simulink model "intelligent_vehicle_example2"  (R2017a)
settings: Solver=VariableStepAuto  StartTime=0.0  StopTime=10.0  RelTol=1e-3
undefined symbols (not defined in the file or in its folder): b1, b2, K1, K2, M1, M2
settings Model: Creator=edward  LastModifiedBy=edward

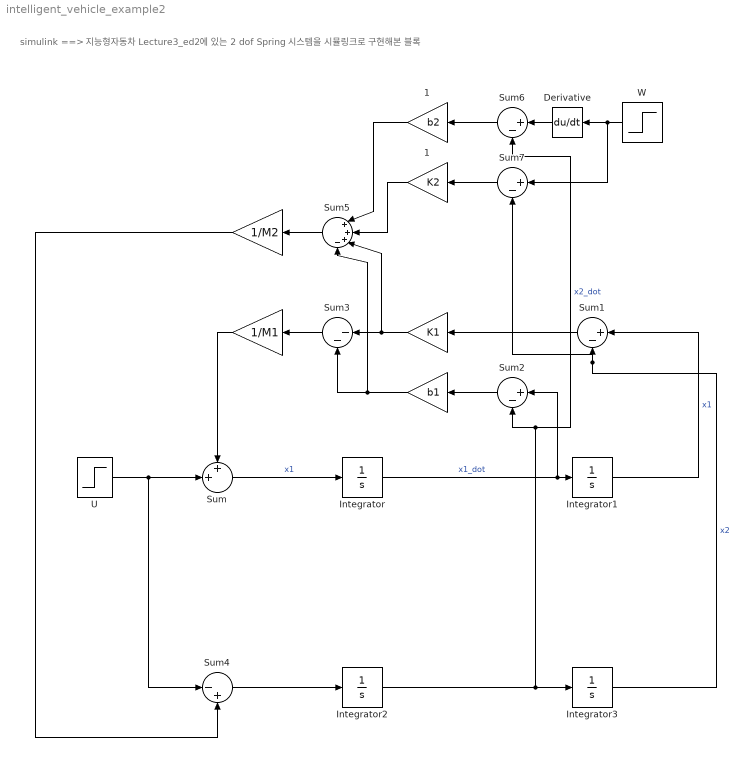
== system intelligent_vehicle_example2 ==
  note: simulink ==> 지능형자동차 Lecture3_ed2에 있는 2 dof Spring 시스템을 시뮬링크로 구현해본 블록
  " " : Gain  Gain=1/M2
  "  " : Gain  Gain=1/M1
  "   " : Gain  Gain=K1
  "    " : Gain  Gain=b1
  "    1" : Gain  Gain=b2
  "   1" : Gain  Gain=K2
  Derivative : Derivative
  Integrator{,1..3} (4 alike) : Integrator
  Sum : Sum  Inputs=++|
  Sum{1..2,6..7} (4 alike) : Sum  Inputs=|+-
  Sum3 : Sum  Inputs=|--
  Sum4 : Sum  Inputs=|-+
  Sum5 : Sum  Inputs=|+++-
  U : Step  SampleTime=0
  W : Step  SampleTime=0
  wires:
  W/1 -> Sum7/1, Derivative/1
  " "/1 -> Sum4/2
  Sum4/1 -> Integrator2/1
  Sum6/1 -> "    1"/1
  Sum1/1 -> "   "/1
  Sum2/1 -> "    "/1
  "  "/1 -> Sum/1
  Sum3/1 -> "  "/1
  Sum7/1 -> "   1"/1
  Derivative/1 -> Sum6/1
  Sum5/1 -> " "/1
  "   "/1 -> Sum5/3, Sum3/1
  "    "/1 -> Sum5/4, Sum3/2
  Integrator2/1 -> Sum6/2, Sum2/2, Integrator3/1  "x2_dot"
  "    1"/1 -> Sum5/1
  Integrator3/1 -> Sum7/2, Sum1/2  "x2"
  U/1 -> Sum4/1, Sum/2
  Integrator1/1 -> Sum1/1  "x1"
  "   1"/1 -> Sum5/2
  Sum/1 -> Integrator/1  "x1"
  Integrator/1 -> Sum2/1, Integrator1/1  "x1_dot"
